simulink model "FluidEnergyBalEx"  (R2015a)
settings: Solver=ode45  StartTime=0.0  StopTime=10.0  RelTol=1e-3
values from neighbouring files (symbols this model uses):
  hc = 10*ones(1,N)    [run_FluidEnergyBalEx.m]
  hd = 10*ones(1,N)    [run_FluidEnergyBalEx.m]
  mdot_bld = [0.02 -0.05]    [run_FluidEnergyBalEx.m]
  mdot_in = 0.1    [run_FluidEnergyBalEx.m]
  T_bld = [550 550]    [run_FluidEnergyBalEx.m]
  T_in = 550    [run_FluidEnergyBalEx.m]
  Tc = linspace(650,1200,N)    [run_FluidEnergyBalEx.m]
  Td = linspace(600,750,N)    [run_FluidEnergyBalEx.m]
libraries: lib_Convection_FluidEnergyBalance x1
settings Model: Creator=jlkratz  LastModifiedBy=jlkratz

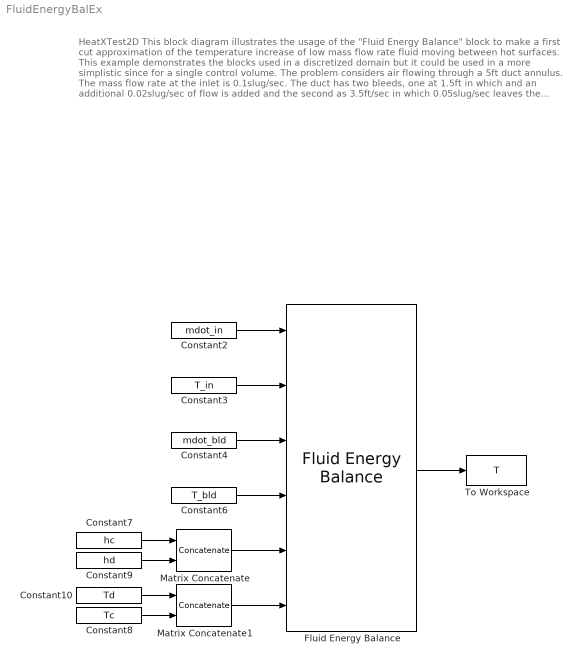
== system FluidEnergyBalEx ==
  note: HeatXTest2D
      |
      | This block diagram illustrates the usage of the "Fluid Energy Balance" block to make a first cut
      | approximation of the temperature increase of low mass flow rate fluid moving between hot surfaces.
      | This example demonstrates the blocks used in a discretized domain but it could be used in a more
      | simplistic since for a single control volume.
      |
      | The problem considers air flowing through a 5ft duct annulus. The mass flow rate at the inlet is 0.1slug/sec.
      | The duct has two bleeds, one at 1.5ft in which and an additional 0.02slug/sec of flow is added and the second
      | as 3.5ft/sec in which 0.05slug/sec leaves the duct. The temperature of the air source entering the duct as 550R.
      | The inner surface changes radius linearly from 0.625ft to 1.15ft and the outer surface has a radius of 1.25ft. The
      | temperature of the inner surface varies linearly from 650R to 1200R and the outer surface varies linearly from
      | 600R to 750R. The heat transfer coefficient between the fluid and both surfaces is assumed to be constant at
      | 10ft-lbf/(sec-ft^2-R). The objective is to approximate the temperature profile of the fluid along the length of the
      | duct.
  Constant10 : Constant  Value=Td
  Constant2 : Constant  Value=mdot_in
  Constant3 : Constant  Value=T_in
  Constant4 : Constant  Value=mdot_bld
  Constant6 : Constant  Value=T_bld
  Constant7 : Constant  Value=hc
  Constant8 : Constant  Value=Tc
  Constant9 : Constant  Value=hd
  Fluid Energy Balance : lib_Convection_FluidEnergyBalance/Fluid Energy Balance  x_M=x  As_M=Ac  Blds_M=on  xbld_M=x_bld  CpData_M=CpData_M  TData_M=TData_M  Tin0_M=T_in  BN_M=double(gcb)
  Matrix Concatenate : Concatenate  Mode=Multidimensional array  ConcatenateDimension=2
  Matrix Concatenate1 : Concatenate  Mode=Multidimensional array  ConcatenateDimension=2
  To Workspace : ToWorkspace  VariableName=T  SampleTime=-1
  wires:
  Constant2/1 -> Fluid Energy Balance/1
  Constant3/1 -> Fluid Energy Balance/2
  Constant4/1 -> Fluid Energy Balance/3
  Constant6/1 -> Fluid Energy Balance/4
  Fluid Energy Balance/1 -> To Workspace/1
  Matrix Concatenate/1 -> Fluid Energy Balance/5
  Matrix Concatenate1/1 -> Fluid Energy Balance/6
  Constant8/1 -> Matrix Concatenate1/2
  Constant10/1 -> Matrix Concatenate1/1
  Constant9/1 -> Matrix Concatenate/2
  Constant7/1 -> Matrix Concatenate/1
